simulink model "test_mftyre_cpi"  (Simulink 4.1.1)
settings: Solver=ode4  SolverMode=SingleTasking  StartTime=0.0  StopTime=2*pi  FixedStep=0.02  MaxStep=0.02  RelTol=1e-5  AbsTol=1e-5
undefined symbols (not defined in the file or in its folder): mfread
libraries: simulink3 x2, dtlib x1
settings Model: LastModifiedBy=besselink  InitialStep=0.01  LimitDataPoints=off  ExtModeTrigMode=oneshot  ExtModeArmWhenConnect=off

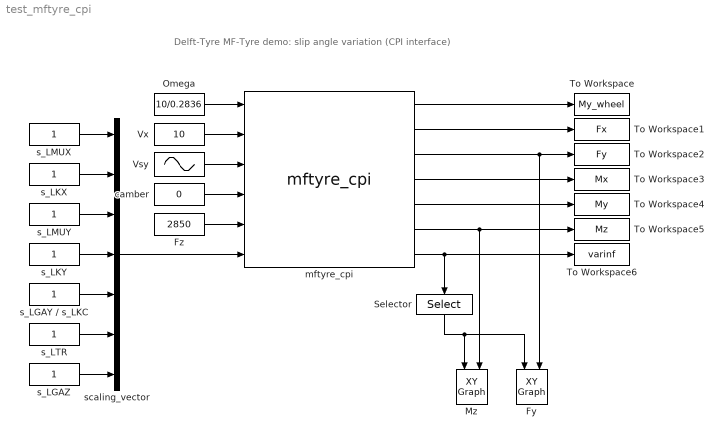
== system test_mftyre_cpi ==
  note: Delft-Tyre MF-Tyre demo: slip angle variation (CPI interface)
  Fy : simulink3/Sinks/XY Graph  Orientation=down  xmin=-0.3  xmax=0.3  ymin=-3500  ymax=3500  st=-1
  Fz : Constant  Value=2850
  Mz : simulink3/Sinks/XY Graph  Orientation=down  xmin=-0.3  xmax=0.3  ymin=-50  ymax=50  st=-1
  Omega : Constant  Value=10/0.2836
  Selector : Selector  Orientation=down  InputType=Vector  ElementSrc=Internal  Elements=1  RowSrc=Internal  Rows=1  ColumnSrc=Internal  Columns=1  InputPortWidth=40
  To Workspace : ToWorkspace  VariableName=My_wheel  SampleTime=-1  SaveFormat=Array
  To Workspace1 : ToWorkspace  VariableName=Fx  SampleTime=-1  SaveFormat=Array
  To Workspace2 : ToWorkspace  VariableName=Fy  SampleTime=-1  SaveFormat=Array
  To Workspace3 : ToWorkspace  VariableName=Mx  SampleTime=-1  SaveFormat=Array
  To Workspace4 : ToWorkspace  VariableName=My  SampleTime=-1  SaveFormat=Array
  To Workspace5 : ToWorkspace  VariableName=Mz  SampleTime=-1  SaveFormat=Array
  To Workspace6 : ToWorkspace  VariableName=varinf  SampleTime=-1  SaveFormat=Array
  Vsy : Sin  SineType=Time-based  Amplitude=5  Bias=0  Frequency=1  Phase=0  Samples=10  SampleTime=0  Offset=0
  Vx : Constant  Value=10
  camber : Constant  Value=0
  mftyre_cpi : dtlib/mftyre_cpi  idtyre=1  typarr=mfread('mft_car175_70R13.tir')  use_mode=4
  s_LGAY / s_LKC : Constant  Value=1
  s_LGAZ : Constant  Value=1
  s_LKX : Constant  Value=1
  s_LKY : Constant  Value=1
  s_LMUX : Constant  Value=1
  s_LMUY : Constant  Value=1
  s_LTR : Constant  Value=1
  scaling_vector : Mux  Inputs=7
  wires:
  Omega/1 -> mftyre_cpi/1
  Vx/1 -> mftyre_cpi/2
  Vsy/1 -> mftyre_cpi/3
  camber/1 -> mftyre_cpi/4
  Fz/1 -> mftyre_cpi/5
  scaling_vector/1 -> mftyre_cpi/6
  s_LMUX/1 -> scaling_vector/1
  s_LKX/1 -> scaling_vector/2
  s_LMUY/1 -> scaling_vector/3
  s_LKY/1 -> scaling_vector/4
  s_LGAY / s_LKC/1 -> scaling_vector/5
  s_LTR/1 -> scaling_vector/6
  s_LGAZ/1 -> scaling_vector/7
  mftyre_cpi/7 -> To Workspace6/1, Selector/1
  mftyre_cpi/6 -> To Workspace5/1, Mz/2
  mftyre_cpi/1 -> To Workspace/1
  mftyre_cpi/2 -> To Workspace1/1
  mftyre_cpi/4 -> To Workspace3/1
  mftyre_cpi/5 -> To Workspace4/1
  mftyre_cpi/3 -> To Workspace2/1, Fy/2
  Selector/1 -> Mz/1, Fy/1
